simulink model "BACKSTEPPING_CORREGIDO"  (R2024a)
settings: Solver=VariableStepAuto  StartTime=0.0  StopTime=50  RelTol=1e-3
settings Model: Creator=VICTUS  LastModifiedBy=VICTUS

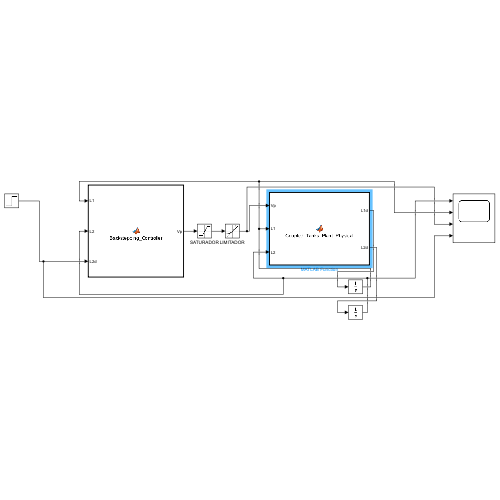
[thumbnail: Simulink's stored preview of the top-level diagram]
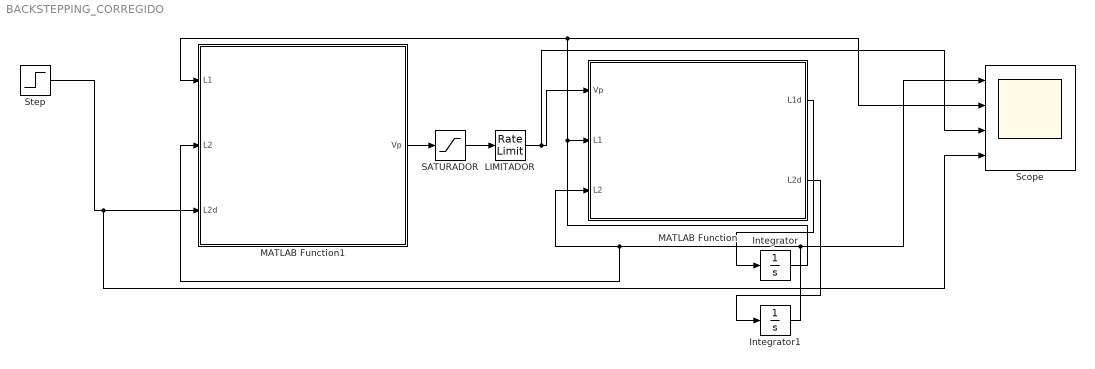
== system BACKSTEPPING_CORREGIDO ==
  Integrator : Integrator
  Integrator1 : Integrator
  LIMITADOR : RateLimiter  RisingSlewLimit=50  FallingSlewLimit=-50  SampleTimeMode=inherited
  MATLAB Function : MATLAB Function  TreatAsAtomicUnit=on
  MATLAB Function1 : MATLAB Function  TreatAsAtomicUnit=on
  SATURADOR : Saturate  UpperLimit=22  LowerLimit=0
  Scope : Scope  NumInputPorts=4
  Step : Step  Time=0  After=10  SampleTime=0.001
  wires:
  Integrator1/1 -> MATLAB Function1/2(L2), MATLAB Function/3(L2), Scope/1
  MATLAB Function/1(L1d) -> Integrator/1
  Integrator/1 -> Scope/2, MATLAB Function1/1(L1), MATLAB Function/2(L1)
  MATLAB Function/2(L2d) -> Integrator1/1
  Step/1 -> Scope/4, MATLAB Function1/3(L2d)
  MATLAB Function1/1(Vp) -> SATURADOR/1
  SATURADOR/1 -> LIMITADOR/1
  LIMITADOR/1 -> Scope/3, MATLAB Function/1(Vp)

== matlab function BACKSTEPPING_CORREGIDO/MATLAB Function1 ==
  data: L1 input; Vp output; L2 input; L2d input
function Vp = Backstepping_Controller(L1, L2, L2d)


%% ===== PARÁMETROS FÍSICOS DEL SISTEMA =====
dt1 = 4.445;   % diámetro tanque 1 [cm]
dt2 = 4.445;   % diámetro tanque 2 [cm]
d01 = 0.635;   % diámetro orificio tanque 1 [cm]
d02 = 0.47625; % diámetro orificio tanque 2 [cm]
At1 = pi*(dt1^2)/4;   % área transversal tanque 1 [cm²]
At2 = pi*(dt2^2)/4;   % área transversal tanque 2 [cm²]
Ao1 = pi*(d01^2)/4;   % área orificio tanque 1 [cm²]
Ao2 = pi*(d02^2)/4;   % área orificio tanque 2 [cm²]
Kp = 3.3;              % constante de bomba [cm³/s/V]
g  = 981;              % gravedad [cm/s²]

%% ===== CÁLCULO DE CONSTANTES EQUIVALENTES =====
k1 = Kp / At1;
k2 = (Ao1 * sqrt(2*g)) / At1;
k3 = (Ao1 * sqrt(2*g)) / At2;
k4 = (Ao2 * sqrt(2*g)) / At2;

%% ===== PARÁMETROS DE CONTROL (MODIFICADOS) =====
c1 = 0.5;  % Reducidos para mayor suavidad
c2 = 1.5;

%% ===== CÁLCULO DE ERRORES =====
z1 = L2 - L2d;  % error de seguimiento

% Control virtual (α₁) con protección contra división por cero
if L2 <= 0
    alpha1 = (1/k3) * (- c1*z1);
else
    alpha1 = (1/k3) * (k4*sqrt(L2) - c1*z1);
end

% Derivada parcial ∂α₁/∂L₂ con protección
if L2 <= 0
    dalpha_dL2 = (1/k3) * (- c1);
else
    dalpha_dL2 = (1/k3) * (k4/(2*sqrt(L2)) - c1);
end

% Segundo error
if L1 <= 0
    z2 = 0 - alpha1;  % Evitar sqrt de negativo
else
    z2 = sqrt(L1) - alpha1;
end

%% ===== LEY DE CONTROL BACKSTEPPING =====
if L1 <= 0
    % Caso especial cuando L1 es muy pequeño
    Vp = 0.001;  % Valor mínimo de seguridad
else
    % Cálculo completo del control
    term1 = -c2*z2;
    term2 = -k3*z1;
    term3 = (k2/2);
    
    if L2 <= 0
        term4 = dalpha_dL2*(k3*sqrt(L1));
    else
        term4 = dalpha_dL2*(k3*sqrt(L1) - k4*sqrt(L2));
    end
    
    Vp = ((2*sqrt(L1)/k1) * (term1 + term2 + term3 + term4));
end


end

== matlab function BACKSTEPPING_CORREGIDO/MATLAB Function ==
  data: Vp input; L1d output; L2d output; L1 input; L2 input
function [L1d, L2d] = Coupled_Tanks_Plant_Physical(Vp,L1, L2)
% Modelo no lineal simplificado de tanques acoplados Quanser

dt1 = 4.445; dt2 = 4.445;
d01 = 0.635; d02 = 0.47625;
At1 = pi*(dt1^2)/4;  At2 = pi*(dt2^2)/4;
Ao1 = pi*(d01^2)/4;  Ao2 = pi*(d02^2)/4;
Kp = 3.3;  g = 981;


Fin = Kp * Vp;
Fout1 = Ao1 * sqrt(2*g*L1);
Fout2 = Ao2 * sqrt(2*g*L2);
F12 = Fout1;

L1d = (Fin - Fout1) / At1;
L2d = (F12 - Fout2) / At2;
end
